simulink model "acquisition_voix"  (Simulink 7.4)
settings: Solver=ode45  StartTime=0.0  StopTime=inf  RelTol=1e-3
values from neighbouring files (symbols this model uses):
  D = ones(n,m) * realmax    [distance_dtw.m]
libraries: dspsnks4 x2, dspwin32 x1
settings Model: Creator=Nayve  LastModifiedBy=Nayve
settings DataIOCC: SignalLoggingName=sigsOut
settings DebuggingCC: SaveWithParameterizedLinksMsg=none  SignalResolutionControl=TryResolveAllWithWarning  SolverPrmCheckMsg=none  MultiTaskDSMMsg=warning  MultiTaskCondExecSysMsg=none  StrictBusMsg=None
settings HardwareCC: TargetUnknown=on
settings RTWCC: IncludeERTFirstTime=on

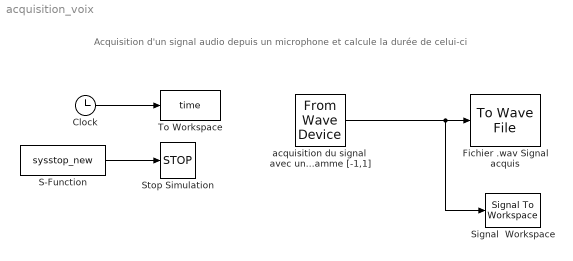
== system acquisition_voix ==
  note: Acquisition d'un signal audio depuis un microphone
      | et calcule la durée de celui-ci
  Clock : Clock
      settings: Decimation=10
  Fichier .wav Signal acquis : dspsnks4/To Wave File  filename=voix.wav  sampleWidth=32  MinNumSamples=256
  S-Function : S-Function  FunctionName=sysstop_new  EnableBusSupport=off
  Signal  Workspace : dspsnks4/Signal To Workspace  SystemSampleTime=-1  VariableName=voix  FrameMode=Concatenate frames (2-D array)
      settings: FixptAsFi=off
  Stop Simulation : Stop
  To Workspace : ToWorkspace  VariableName=time  SampleTime=-1  SaveFormat=Structure With Time
      settings: MaxDataPoints=1
  acquisition du signal  avec un microphone Gamme [-1,1] : dspwin32/From Wave Device  SampleRate=8000  UserRate=16000  SampleWidth=16  Stereo=off  SamplesPerFrame=80  QueueDuration=1  useDefaultDevice=on  userDeviceID=<empty>  dType=double
  wires:
  acquisition du signal  avec un microphone Gamme [-1,1]/1 -> Fichier .wav Signal acquis/1, Signal  Workspace/1
  S-Function/1 -> Stop Simulation/1
  Clock/1 -> To Workspace/1
